simulink model "q10"  (R2020a)
settings: Solver=VariableStepAuto  StartTime=0.0  StopTime=10.0  RelTol=1e-3
libraries: simulink x1
settings Model: Creator=kiran  LastModifiedBy=kiran

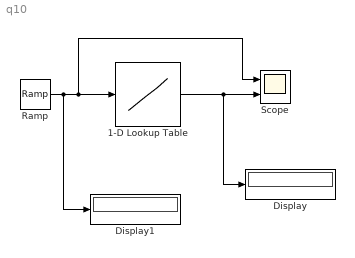
== system q10 ==
  1-D Lookup Table : Lookup_n-D  NumberOfTableDimensions=1  BreakpointsForDimension1=[0 0.1 0.2 0.3 0.4 0.6 0.8 1.0 1.2 1.4 1.6 1.8 2.0 2.2 2.4]  Table=[0 0 0 0 0.5 1 2 3 5 7.5 10 15 20 25 30]  InternalRulePriority=Speed  RndMeth=Simplest  InputSameDT=on
  Display : Display
  Display1 : Display
  Ramp : simulink/Sources/Ramp  slope=1  start=0  InitialOutput=0
  Scope : Scope  NumInputPorts=2
  wires:
  1-D Lookup Table/1 -> Display/1, Scope/2
  Ramp/1 -> Display1/1, Scope/1, 1-D Lookup Table/1
